simulink model "example4"  (R2019b)
settings: Solver=ode4  StartTime=0.0  StopTime=4  RelTol=1e-3
settings Model: Creator=davis  LastModifiedBy=davis

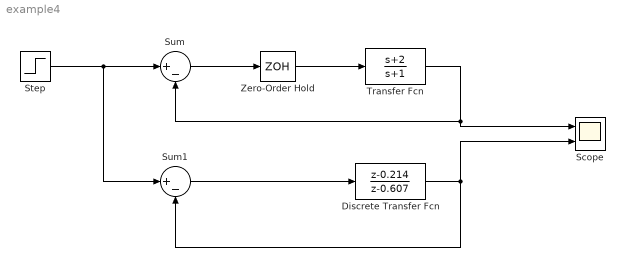
== system example4 ==
  Discrete Transfer Fcn : DiscreteTransferFcn  Numerator=[1 -0.214]  Denominator=[1 -0.607]  SampleTime=0.5
  Scope : Scope  NumInputPorts=2
  Step : Step  Time=0  SampleTime=0
  Sum : Sum  Inputs=|+-
  Sum1 : Sum  Inputs=|+-
  Transfer Fcn : TransferFcn  Numerator=[1 2]  Denominator=[1 1]
  Zero-Order Hold : ZeroOrderHold  SampleTime=0.5
  wires:
  Step/1 -> Sum1/1, Sum/1
  Sum/1 -> Zero-Order Hold/1
  Zero-Order Hold/1 -> Transfer Fcn/1
  Transfer Fcn/1 -> Scope/1, Sum/2
  Sum1/1 -> Discrete Transfer Fcn/1
  Discrete Transfer Fcn/1 -> Scope/2, Sum1/2
